simulink model "Practica2p220"  (R2014b)
settings: Solver=ode45  StartTime=0.0  StopTime=100.0  MaxStep=0.1  RelTol=1e-3
settings Model: Creator=usuario_local  LastModifiedBy=usuario_local

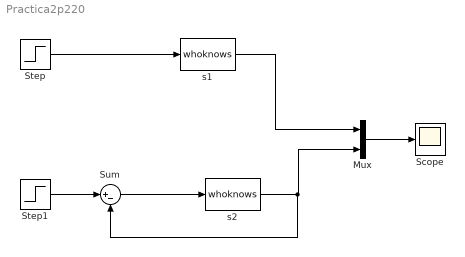
== system Practica2p220 ==
  Mux : Mux  Inputs=2
  Scope : Scope
      settings: YMin=0  YMax=1.2
  Step : Step  SampleTime=0
  Step1 : Step  SampleTime=0
  Sum : Sum  Inputs=|+-
  s1 : M-S-Function  FunctionName=whoknows  Parameters=L, P1, P2, T, R  mask{L=8, P1=1, P2=7, T=2, R=0}
      mask prompts: L "Laboratorio"; P1 "Primer digito del Puesto"; P2 "Segundo digito del Puesto"; T "Tipo de Planta"; R "Ruido"
      mask Display: disp('Sistema')
  s2 : M-S-Function  FunctionName=whoknows  Parameters=L, P1, P2, T, R  mask{L=8, P1=1, P2=7, T=2, R=0}
      mask prompts: L "Laboratorio"; P1 "Primer digito del Puesto"; P2 "Segundo digito del Puesto"; T "Tipo de Planta"; R "Ruido"
      mask Display: disp('Sistema')
  wires:
  Step/1 -> s1/1
  Step1/1 -> Sum/1
  s1/1 -> Mux/1
  Mux/1 -> Scope/1
  Sum/1 -> s2/1
  s2/1 -> Sum/2, Mux/2
